simulink model "ADP_demo"  (R2013a)
settings: Solver=ode45  StartTime=0.0  StopTime=10  FixedStep=0.01  MaxStep=0.01  RelTol=1e-3
libraries: ADPLib x1, simulink x1
settings Model: Creator=Yuri  LastModifiedBy=Yuri
settings SolverCC: ZeroCrossControl=EnableAll  ZeroCrossAlgorithm=Adaptive
settings DebuggingCC: AlgebraicLoopMsg=none  UnderspecifiedInitializationDetection=Simplified  MergeDetectMultiDrivingBlocksExec=error  MultiTaskDSMMsg=none  StateNameClashWarn=none
settings RTWCC: GenCodeOnly=on
settings GRTTargetCC: CodeReplacementLibrary=C89/C90 (ANSI)

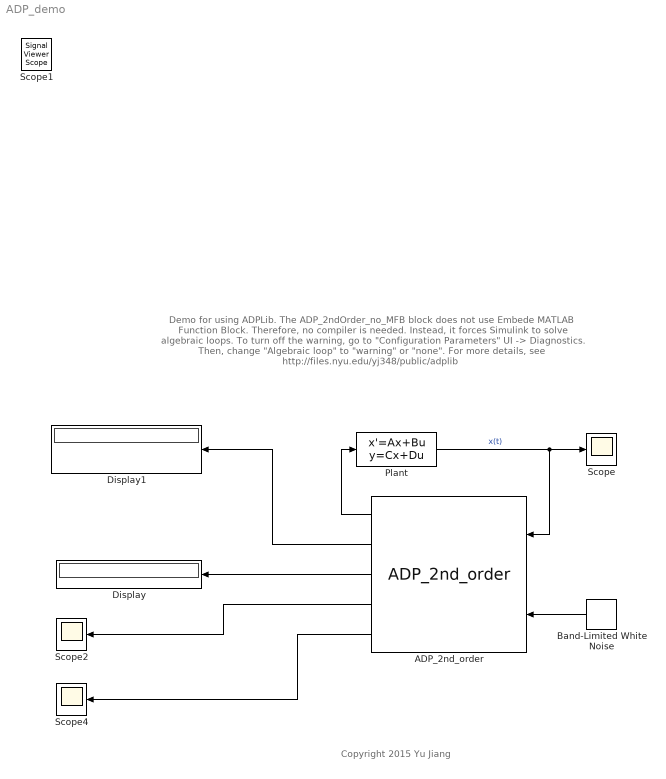
== system ADP_demo ==
  note: Copyright 2015 Yu Jiang
  note: Demo for using ADPLib.
      | The ADP_2ndOrder_no_MFB block does not use Embede MATLAB Function Block.
      | Therefore, no compiler is needed. Instead, it forces Simulink to solve algebraic loops.
      | To turn off the warning, go to "Configuration Parameters"  UI -> Diagnostics.
      | Then, change "Algebraic loop" to "warning" or "none".
      |
      | For more details, see
      | http://files.nyu.edu/yj348/public/adplib
  ADP_2nd_order : ADPLib/ADP_2nd_order  K=[0,0]  Q=eye(2)  R=1  dT=0.1  epsilon=.00001
  Band-Limited White Noise : simulink/Sources/Band-Limited White Noise  Cov=[0.1]  Ts=0.01  seed=[23341]
  Display : Display
  Display1 : Display
  Plant : StateSpace  A=[0 1;-0.2 -0.1];  B=[0.03;.6];  C=eye(2)  D=zeros(2,1)  X0=[1;2]
  Scope : Scope
      settings: TimeRange=10  YMin=-0.7  YMax=0.5
  Scope2 : Scope
      settings: SaveName=ScopeData2
  Scope4 : Scope
      settings: SaveName=ScopeData3
  Scope1 : SignalViewerScope  IOType=viewer  RefreshTime=0.035000
      settings: SaveName=ScopeData2  DataFormat=StructureWithTime
  wires:
  Plant/1 -> ADP_2nd_order/1, Scope/1  "x(t)"
  ADP_2nd_order/1 -> Plant/1
  ADP_2nd_order/2 -> Display1/1
  ADP_2nd_order/3 -> Display/1
  ADP_2nd_order/4 -> Scope2/1
  Band-Limited White Noise/1 -> ADP_2nd_order/2
  ADP_2nd_order/5 -> Scope4/1
